simulink model "TEST_O_sim_NO_3D"  (R2013a)
settings: Solver=ode45  StartTime=0.0  StopTime=10.0  RelTol=1e-3
values from neighbouring files (symbols this model uses):
  Mu = (3.9856e+14)    (= 398560000000000)    [ATV_laplace_potentials_test0.m]    (also in CW_anlytical.m; Controlled_motion_test1.m; EOS_test.m; Hill_TEST.m)
  R_0c = (R_0t+rand(3,1)*0.25*1e2)    [ATV_laplace_potentials_test0.m]    (also in CW_anlytical.m = [R_C;0;0]; Controlled_motion_test1.m = (R_0t+X_obs+rand(3,1)*0.25*1e2); Hill_TEST.m = (R_0t-rand(3,1)*0.5*1e2); Hill_TEST_INTEGR.m = (R_0t-[d_TC;0;0]))
  R_0t = [R_T;0;0]    [CW_anlytical.m]    (also in Controlled_motion_test1.m = [(r_Earth+h_orb);0;0]; EOS_test.m = [(r_Earth+h_orb);0;0]; Hill_TEST.m = [(r_Earth+h_orb);0;0]; Hill_TEST_INTEGR.m = [(r_Earth+h_orb);0;0])
  V_0c = (V_0t+rand(3,1)*0.5*1e-1)    [ATV_laplace_potentials_test0.m]    (also in CW_anlytical.m = [0;sqrt(Mu/norm(R_0c));0]; Controlled_motion_test1.m = (V_0t-rand(3,1)*0.25*1e-2); Hill_TEST.m; Hill_TEST_INTEGR.m = [0;omega*R_C;0])
  V_0t = [0;sqrt(Mu/(r_Earth+h_orb));0]    [CW_anlytical.m]    (also in Controlled_motion_test1.m; EOS_test.m; Hill_TEST.m; Hill_TEST_INTEGR.m)
undefined symbols (not defined in the file or in its folder): r_0, v_0
settings Model: Creator=teo  LastModifiedBy=teo

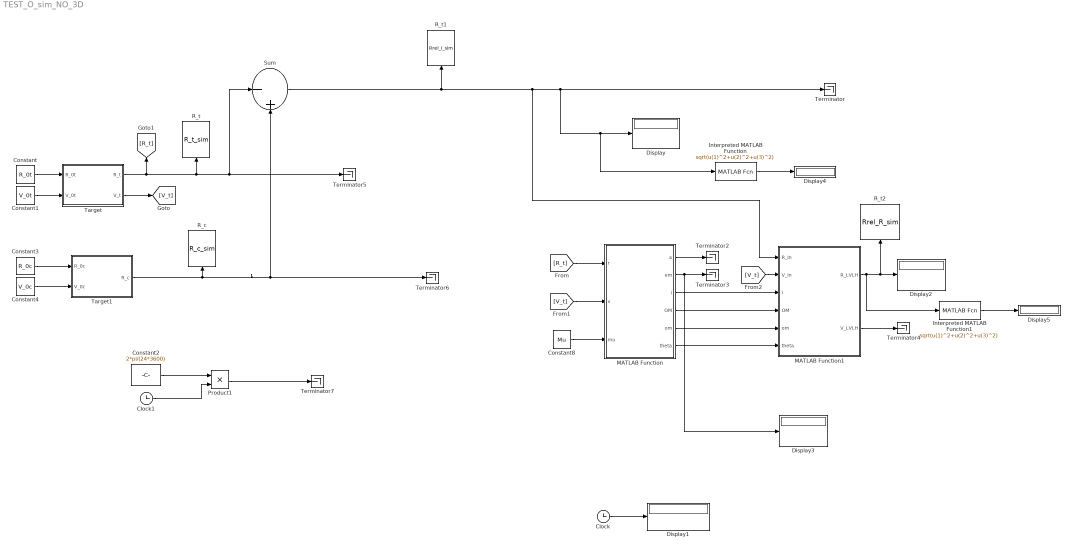
== system TEST_O_sim_NO_3D ==
  Clock : Clock
  Clock1 : Clock
  Constant : Constant  Value=R_0t  VectorParams1D=off
  Constant1 : Constant  Value=V_0t  VectorParams1D=off
  Constant2 : Constant  Value=2*pi/(24*3600)
  Constant3 : Constant  Value=R_0c  VectorParams1D=off
  Constant4 : Constant  Value=V_0c  VectorParams1D=off
  Constant8 : Constant  Value=Mu  VectorParams1D=off
  Display{,1..5} (6 alike) : Display
  Interpreted MATLAB Function : MATLABFcn  MATLABFcn=sqrt(u(1)^2+u(2)^2+u(3)^2)
  Interpreted MATLAB Function1 : MATLABFcn  MATLABFcn=sqrt(u(1)^2+u(2)^2+u(3)^2)
  MATLAB Function : Subsystem  TreatAsAtomicUnit=on
  MATLAB Function1 : Subsystem  TreatAsAtomicUnit=on
  Product1 : Product
  R_c : ToWorkspace  VariableName=R_c_sim  SampleTime=-1  SaveFormat=Structure With Time
  R_t : ToWorkspace  VariableName=R_t_sim  SampleTime=-1  SaveFormat=Structure With Time
  R_t1 : ToWorkspace  VariableName=Rrel_I_sim  SampleTime=-1  SaveFormat=Structure With Time
  R_t2 : ToWorkspace  VariableName=Rrel_R_sim  SampleTime=-1  SaveFormat=Structure With Time
  Sum : Sum  Inputs=|-+
  Target : Subsystem
  Target1 : Subsystem
  Terminator{,2..7} (7 alike) : Terminator
  wires:
  Constant2/1 -> Product1/1
  Product1/1 -> Terminator7/1
  Clock1/1 -> Product1/2
  Target/1(R_t) -> [R_t], Sum/1, Terminator5/1, R_t/1
  Constant/1 -> Target/1(R_0t)
  Constant1/1 -> Target/2(V_0t)
  Target1/1(R_c) -> Sum/2, Terminator6/1, R_c/1
  Constant3/1 -> Target1/1(R_0c)
  Constant4/1 -> Target1/2(V_0c)
  Clock/1 -> Display1/1
  Target/2("V_t ") -> [V_t]
  [V_t] -> MATLAB Function/2(v)
  [R_t] -> MATLAB Function/1(r)
  Constant8/1 -> MATLAB Function/3(mu)
  MATLAB Function/1(a) -> Terminator2/1
  MATLAB Function/2(em) -> Display3/1, Terminator3/1
  MATLAB Function/3(i) -> MATLAB Function1/3(i)
  MATLAB Function/4(OM) -> MATLAB Function1/4(OM)
  MATLAB Function/5(om) -> MATLAB Function1/5(om)
  MATLAB Function/6(theta) -> MATLAB Function1/6(theta)
  MATLAB Function1/2(V_LVLH) -> Terminator4/1
  [V_t] -> MATLAB Function1/2(V_In)
  Interpreted MATLAB Function/1 -> Display4/1
  MATLAB Function1/1(R_LVLH) -> Interpreted MATLAB Function1/1, Display2/1, R_t2/1
  Interpreted MATLAB Function1/1 -> Display5/1
  Sum/1 -> R_t1/1, Terminator/1, Interpreted MATLAB Function/1, Display/1, MATLAB Function1/1(R_In)

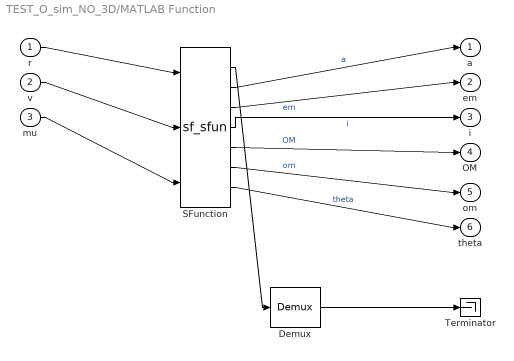
== system TEST_O_sim_NO_3D/MATLAB Function ==
  r : Inport
  v : Inport  Port=2
  mu : Inport  Port=3
  " Demux " : Demux  Outputs=1
  " SFunction " : S-Function  Tag=Stateflow S-Function TEST_0_sim 2  FunctionName=sf_sfun  PortCounts=[3 7]  EnableBusSupport=on
  " Terminator " : Terminator
  a : Outport
  em : Outport  Port=2
  i : Outport  Port=3
  OM : Outport  Port=4
  om : Outport  Port=5
  theta : Outport  Port=6
  wires:
  r/1 -> " SFunction "/1
  v/1 -> " SFunction "/2
  mu/1 -> " SFunction "/3
  " SFunction "/2 -> a/1  "a"
  " SFunction "/3 -> em/1  "em"
  " SFunction "/4 -> i/1  "i"
  " SFunction "/5 -> OM/1  "OM"
  " SFunction "/6 -> om/1  "om"
  " SFunction "/7 -> theta/1  "theta"
  " Demux "/1 -> " Terminator "/1
  " SFunction "/1 -> " Demux "/1

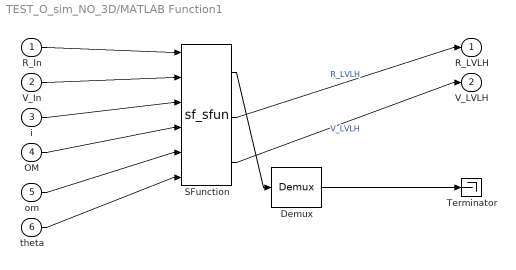
== system TEST_O_sim_NO_3D/MATLAB Function1 ==
  R_In : Inport
  V_In : Inport  Port=2
  i : Inport  Port=3
  OM : Inport  Port=4
  om : Inport  Port=5
  theta : Inport  Port=6
  " Demux " : Demux  Outputs=1
  " SFunction " : S-Function  Tag=Stateflow S-Function TEST_0_sim 1  FunctionName=sf_sfun  PortCounts=[6 3]  EnableBusSupport=on
  " Terminator " : Terminator
  R_LVLH : Outport
  V_LVLH : Outport  Port=2
  wires:
  R_In/1 -> " SFunction "/1
  V_In/1 -> " SFunction "/2
  i/1 -> " SFunction "/3
  OM/1 -> " SFunction "/4
  om/1 -> " SFunction "/5
  theta/1 -> " SFunction "/6
  " SFunction "/2 -> R_LVLH/1  "R_LVLH"
  " SFunction "/3 -> V_LVLH/1  "V_LVLH"
  " Demux "/1 -> " Terminator "/1
  " SFunction "/1 -> " Demux "/1

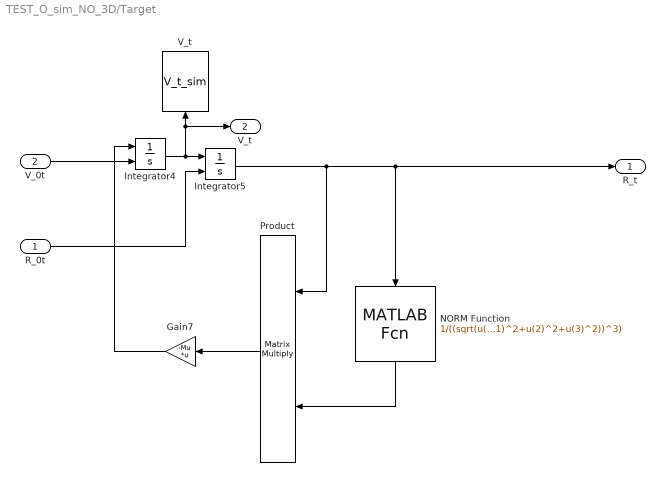
== system TEST_O_sim_NO_3D/Target ==
  R_0t : Inport
  V_0t : Inport  Port=2
  Gain7 : Gain  Gain=-Mu  Multiplication=Matrix(K*u)
  Integrator4 : Integrator  InitialConditionSource=external  InitialCondition=v_0
  Integrator5 : Integrator  InitialConditionSource=external  InitialCondition=r_0
  NORM Function : MATLABFcn  MATLABFcn=1/((sqrt(u(1)^2+u(2)^2+u(3)^2))^3)  OutputDimensions=1
  Product : Product  Multiplication=Matrix(*)
  V_t : ToWorkspace  VariableName=V_t_sim  SampleTime=-1  SaveFormat=Structure With Time
  R_t : Outport
  "V_t " : Outport  Port=2
  wires:
  Integrator5/1 -> R_t/1, NORM Function/1, Product/1
  Integrator4/1 -> Integrator5/1, "V_t "/1, V_t/1
  Gain7/1 -> Integrator4/1
  Product/1 -> Gain7/1
  NORM Function/1 -> Product/2
  V_0t/1 -> Integrator4/2
  R_0t/1 -> Integrator5/2

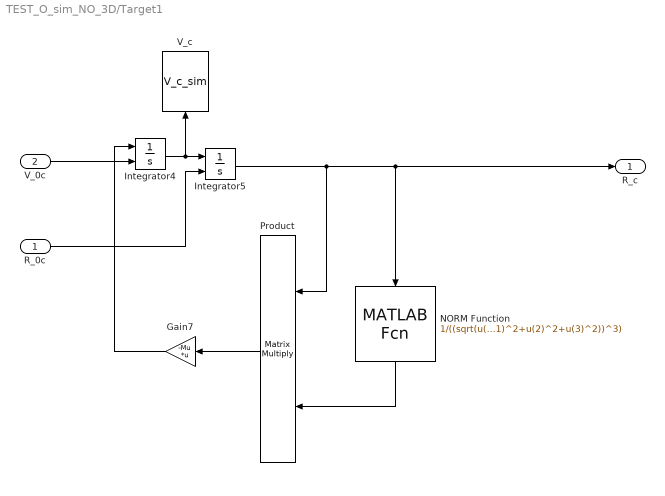
== system TEST_O_sim_NO_3D/Target1 ==
  R_0c : Inport
  V_0c : Inport  Port=2
  Gain7 : Gain  Gain=-Mu  Multiplication=Matrix(K*u)
  Integrator4 : Integrator  InitialConditionSource=external  InitialCondition=v_0
  Integrator5 : Integrator  InitialConditionSource=external  InitialCondition=r_0
  NORM Function : MATLABFcn  MATLABFcn=1/((sqrt(u(1)^2+u(2)^2+u(3)^2))^3)  OutputDimensions=1
  Product : Product  Multiplication=Matrix(*)
  V_c : ToWorkspace  VariableName=V_c_sim  SampleTime=-1  SaveFormat=Structure With Time
  R_c : Outport
  wires:
  Integrator5/1 -> R_c/1, NORM Function/1, Product/1
  Integrator4/1 -> Integrator5/1, V_c/1
  Gain7/1 -> Integrator4/1
  Product/1 -> Gain7/1
  NORM Function/1 -> Product/2
  V_0c/1 -> Integrator4/2
  R_0c/1 -> Integrator5/2
